simulink model "sensorMCUSlugsMKII"  (Simulink 7.8)
settings: Solver=FixedStepDiscrete  SolverMode=SingleTasking  StartTime=0.0  StopTime=inf  FixedStep=0.01  RelTol=1e-3
InitFcn:
  | mcuInit
values from neighbouring files (symbols this model uses):
  apSampleTime = 0.01    [mcuInit.m]
  T = 0.01    [mcuInit.m]
undefined symbols (not defined in the file or in its folder): accBiasRateLimit, barAdjust, baroCutoff, baroCutTemp, baroOffset, baroScale, barTGain1, barTGain2, barTMean1, barTMean2, baseHeight, baseTemp, cubeAccelGain16405, cubeGyroGain16405, cubeMagGain16405, DiscIntNeverNeededParam, Function_Update, gaind, getCubeData, getGpsMainData, getGPSRawData, getGpsUbloxMainData, getGSLocation, gpsParse, gyroBiasRateLimit, hil_getEuler, hil_getRates, hil_getRawRead, hil_getVned, hil_getXYZ, hilRead, Init_onlyOnce, Init_Reset, lapseRate, lowRateSensorCutoff, mainSensorCutoff, maxDynPressure, pitAdjust, pitCutTemp, pitotOffset, pitotScale, pitTGain1, pitTGain2, pitTMean1, pitTMean2, polesd, powerOffset, powerScale, pressureSensorCutoff, protDecodeHil, q_quat, scheduleData, sensorMCUInit, spiSend, tempOffset, tempScale, u1, u2, U_comm, updateAirData ... (+14)
libraries: dsPICdrivers x47, simulink x7, aerolibutil x4, aerolibtransform2 x2, dspmtrx3 x2, aerolibconvert2 x2
(part 4 of 4)

== matlab function Sensor Data/Sensor Suite/ADIS16405 Signal Cond /3D Tustin Lowpass, Auto Initial Condition1/Embedded MATLAB Function1 ==
  data: u input double; y output double; T input double; f input double
function y = fcn(u,T,f)
% This block supports an embeddable subset of the MATLAB language.
% See the help menu for details. 

persistent a
persistent b
persistent y_km1
persistent u_km1
if isempty(a)
    %tf = [T*omega/(2+T*omega) T*omega/(2+T*omega)],[1 (T*omega-2)/(T*omega+2)]
    %tf = [a a],[1 -b]
    omega = 2*pi*f;
    a=T*omega/(2+T*omega);
    b=-(T*omega-2)/(T*omega+2);
    y_km1=u;
    u_km1=u;
end

y = a*(u+u_km1)+b*y_km1;
y_km1=y;
u_km1=u;

== matlab function Sensor Data/Sensor Suite/ADIS16405 Signal Cond /3D Tustin Lowpass, Auto Initial Condition1/Embedded MATLAB Function2 ==
  data: u input double; y output double; T input double; f input double
function y = fcn(u,T,f)
% This block supports an embeddable subset of the MATLAB language.
% See the help menu for details. 

persistent a
persistent b
persistent y_km1
persistent u_km1
if isempty(a)
    %tf = [T*omega/(2+T*omega) T*omega/(2+T*omega)],[1 (T*omega-2)/(T*omega+2)]
    %tf = [a a],[1 -b]
    omega = 2*pi*f;
    a=T*omega/(2+T*omega);
    b=-(T*omega-2)/(T*omega+2);
    y_km1=u;
    u_km1=u;
end

y = a*(u+u_km1)+b*y_km1;
y_km1=y;
u_km1=u;

== matlab function Sensor Data/Sensor Suite/ADIS16405 Signal Cond /3D Tustin Lowpass, Auto Initial Condition1/myMux Fun ==
  data: u1 input double; y output double; u2 input double; u3 input double
function y = myMux3(u1, u2, u3)
% This block supports an embeddable subset of the MATLAB language.
% See the help menu for details. 

y = [u1(1); u2(1); u3(1)];

== matlab function Sensor Data/Sensor Suite/Low Pass Filtering,Temperature Compensation and Calibration/Baro Altimeter/Enables/Disables the Computation of initial Baro Bias ==
  data: tOut output double
function tOut = getTIni

persistent aveCount;
persistent tIni;

if isempty(aveCount)
    aveCount =1;
    tIni = 1;
end;

if aveCount < 2500
    aveCount = aveCount + 1;
end

if aveCount == 2500
    tIni =0;
    aveCount = aveCount + 1;
end

tOut = tIni;

%if aveCount > 500
%    tIni = 0;
%end

% if isempty(aveCount)
%     aveCount =1;
%     initBias = [0.0 0.0 0.0]';
% end;
%     
% if (aveCount<10)
%     initBias = initBias+ Raw;
%     bias = initBias/aveCount;
%     aveCount = aveCount +1;
% end;
% 
% if (aveCount == 10)
%     initBias = initBias/(aveCount-1);
%     aveCount = 100;
% end;
% 
% if (aveCount == 100)
%     bias = initBias;
% end;

== matlab function Sensor Data/Sensor Suite/Low Pass Filtering,Temperature Compensation and Calibration/Tustin Lowpass, Auto Initial Condition1/Embedded MATLAB Function ==
  data: u input double; y output double; T input double; f input double
function y = fcn(u,T,f)
% This block supports an embeddable subset of the MATLAB language.
% See the help menu for details. 

persistent a
persistent b
persistent y_km1
persistent u_km1
if isempty(a)
    %tf = [T*omega/(2+T*omega) T*omega/(2+T*omega)],[1 (T*omega-2)/(T*omega+2)]
    %tf = [a a],[1 -b]
    omega = 2*pi*f;
    a=T*omega/(2+T*omega);
    b=-(T*omega-2)/(T*omega+2);
    y_km1=u;
    u_km1=u;
end

y = a*(u+u_km1)+b*y_km1;
y_km1=y;
u_km1=u;

== matlab function Sensor Data/Sensor Suite/Low Pass Filtering,Temperature Compensation and Calibration/Tustin Lowpass, Auto Initial Condition2/Embedded MATLAB Function ==
  data: u input double; y output double; T input double; f input double
function y = fcn(u,T,f)
% This block supports an embeddable subset of the MATLAB language.
% See the help menu for details. 

persistent a
persistent b
persistent y_km1
persistent u_km1
if isempty(a)
    %tf = [T*omega/(2+T*omega) T*omega/(2+T*omega)],[1 (T*omega-2)/(T*omega+2)]
    %tf = [a a],[1 -b]
    omega = 2*pi*f;
    a=T*omega/(2+T*omega);
    b=-(T*omega-2)/(T*omega+2);
    y_km1=u;
    u_km1=u;
end

y = a*(u+u_km1)+b*y_km1;
y_km1=y;
u_km1=u;

== matlab function Sensor Data/Sensor Suite/Low Pass Filtering,Temperature Compensation and Calibration/Tustin Lowpass, Auto Initial Condition3/Embedded MATLAB Function ==
  data: u input double; y output double; T input double; f input double
function y = fcn(u,T,f)
% This block supports an embeddable subset of the MATLAB language.
% See the help menu for details. 

persistent a
persistent b
persistent y_km1
persistent u_km1
if isempty(a)
    %tf = [T*omega/(2+T*omega) T*omega/(2+T*omega)],[1 (T*omega-2)/(T*omega+2)]
    %tf = [a a],[1 -b]
    omega = 2*pi*f;
    a=T*omega/(2+T*omega);
    b=-(T*omega-2)/(T*omega+2);
    y_km1=u;
    u_km1=u;
end

y = a*(u+u_km1)+b*y_km1;
y_km1=y;
u_km1=u;

== matlab function Sensor Data/Sensor Suite/Low Pass Filtering,Temperature Compensation and Calibration/Tustin Lowpass, Auto Initial Condition4/Embedded MATLAB Function ==
  data: u input double; y output double; T input double; f input double
function y = fcn(u,T,f)
% This block supports an embeddable subset of the MATLAB language.
% See the help menu for details. 

persistent a
persistent b
persistent y_km1
persistent u_km1
if isempty(a)
    %tf = [T*omega/(2+T*omega) T*omega/(2+T*omega)],[1 (T*omega-2)/(T*omega+2)]
    %tf = [a a],[1 -b]
    omega = 2*pi*f;
    a=T*omega/(2+T*omega);
    b=-(T*omega-2)/(T*omega+2);
    y_km1=u;
    u_km1=u;
end

y = a*(u+u_km1)+b*y_km1;
y_km1=y;
u_km1=u;
